simulink model "Inciso2_G2"  (R2023a)
settings: Solver=VariableStepAuto  StartTime=0.0  StopTime=100.0  RelTol=1e-3
settings Model: Creator=Daniela  LastModifiedBy=Daniela

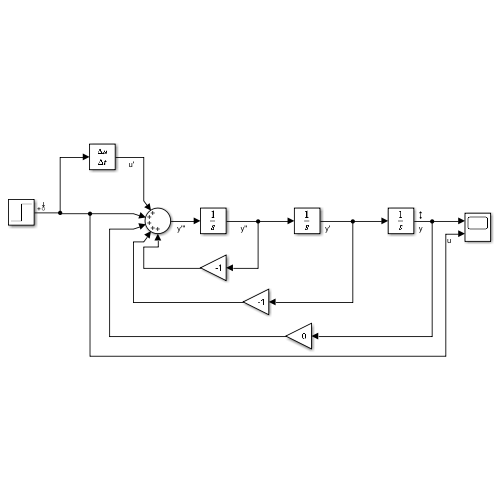
[thumbnail: Simulink's stored preview of the top-level diagram]
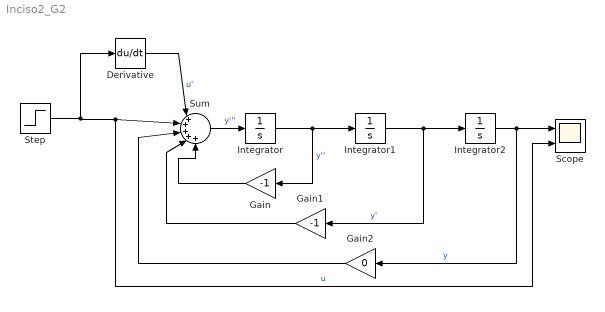
== system Inciso2_G2 ==
  Derivative : Derivative
  Gain : Gain  Gain=-1
  Gain1 : Gain  Gain=-1
  Gain2 : Gain  Gain=0
  Integrator : Integrator
  Integrator1 : Integrator
  Integrator2 : Integrator
  Scope : Scope  NumInputPorts=2
  Step : Step  Time=0  SampleTime=0
  Sum : Sum  Inputs=|+++++
  wires:
  Integrator/1 -> Gain/1, Integrator1/1  "y''"
  Sum/1 -> Integrator/1  "y'''"
  Step/1 -> Derivative/1, Scope/2, Sum/2  "u"
  Integrator1/1 -> Integrator2/1, Gain1/1  "y'"
  Gain/1 -> Sum/5
  Gain1/1 -> Sum/4
  Integrator2/1 -> Gain2/1, Scope/1  "y"
  Gain2/1 -> Sum/3
  Derivative/1 -> Sum/1  "u'"
